simulink model "Ques5_system"  (R2020b)
settings: Solver=VariableStepAuto  StartTime=0.0  StopTime=10.0  RelTol=1e-3
values from neighbouring files (symbols this model uses):
  C = 10*10^-6    (= 1e-05)    [Ques5_code.m]
  R = 10    [Ques5_code.m]
settings Model: Creator=sneha  LastModifiedBy=sneha

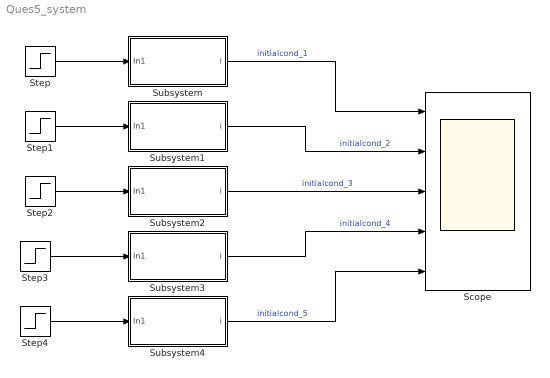
== system Ques5_system ==
  Scope : Scope  NumInputPorts=5
  Step{,1..4} (5 alike) : Step  After=10  SampleTime=0
  Subsystem : Subsystem
  Subsystem1 : Subsystem
  Subsystem2 : Subsystem
  Subsystem3 : Subsystem
  Subsystem4 : Subsystem
  wires:
  Step/1 -> Subsystem/1(In1)
  Subsystem/1(i) -> Scope/1  "initialcond_1"
  Step1/1 -> Subsystem1/1(In1)
  Step2/1 -> Subsystem2/1(In1)
  Step3/1 -> Subsystem3/1(In1)
  Step4/1 -> Subsystem4/1(In1)
  Subsystem1/1(i) -> Scope/2  "initialcond_2"
  Subsystem2/1(i) -> Scope/3  "initialcond_3"
  Subsystem3/1(i) -> Scope/4  "initialcond_4"
  Subsystem4/1(i) -> Scope/5  "initialcond_5"

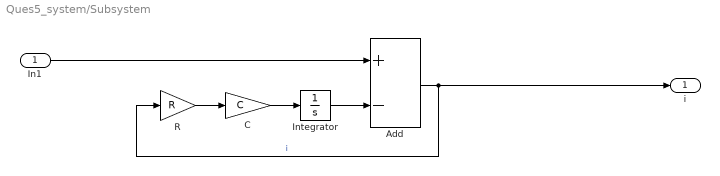
== system Ques5_system/Subsystem ==
  In1 : Inport
  Add : Sum  Inputs=+-
  C : Gain  Gain=C
  Integrator : Integrator  InitialCondition=1
  R : Gain  Gain=R
  i : Outport
  wires:
  R/1 -> C/1
  C/1 -> Integrator/1
  Integrator/1 -> Add/2
  In1/1 -> Add/1
  Add/1 -> i/1, R/1  "i"

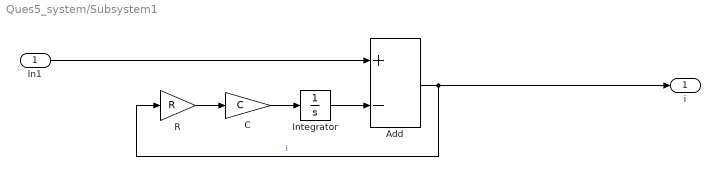
== system Ques5_system/Subsystem1 ==
  In1 : Inport
  Add : Sum  Inputs=+-
  C : Gain  Gain=C
  Integrator : Integrator  InitialCondition=2
  R : Gain  Gain=R
  i : Outport
  wires:
  Add/1 -> R/1, i/1  "i"
  In1/1 -> Add/1
  Integrator/1 -> Add/2
  C/1 -> Integrator/1
  R/1 -> C/1

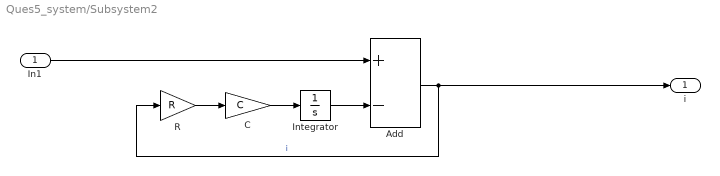
== system Ques5_system/Subsystem2 ==
  In1 : Inport
  Add : Sum  Inputs=+-
  C : Gain  Gain=C
  Integrator : Integrator  InitialCondition=3
  R : Gain  Gain=R
  i : Outport
  wires:
  R/1 -> C/1
  C/1 -> Integrator/1
  Integrator/1 -> Add/2
  In1/1 -> Add/1
  Add/1 -> i/1, R/1  "i"

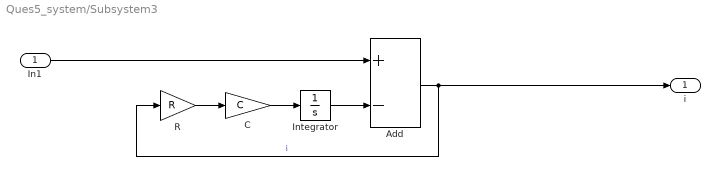
== system Ques5_system/Subsystem3 ==
  In1 : Inport
  Add : Sum  Inputs=+-
  C : Gain  Gain=C
  Integrator : Integrator  InitialCondition=4
  R : Gain  Gain=R
  i : Outport
  wires:
  Add/1 -> R/1, i/1  "i"
  In1/1 -> Add/1
  Integrator/1 -> Add/2
  C/1 -> Integrator/1
  R/1 -> C/1

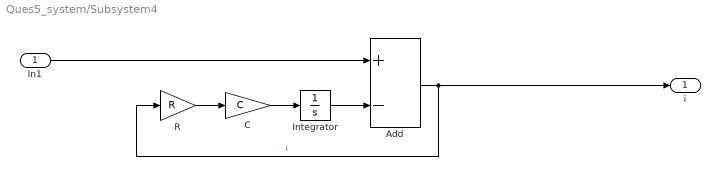
== system Ques5_system/Subsystem4 ==
  In1 : Inport
  Add : Sum  Inputs=+-
  C : Gain  Gain=C
  Integrator : Integrator  InitialCondition=5
  R : Gain  Gain=R
  i : Outport
  wires:
  R/1 -> C/1
  C/1 -> Integrator/1
  Integrator/1 -> Add/2
  In1/1 -> Add/1
  Add/1 -> i/1, R/1  "i"
